simulink model "laboratory2_group2_ME_4212"  (R2024b)
settings: Solver=VariableStepAuto  StartTime=0.0  StopTime=Sim_Time  RelTol=1e-3
undefined symbols (not defined in the file): B1, B2, F, K1, K2, M1, M2
settings Model: Creator=karltzu  LastModifiedBy=karltzu

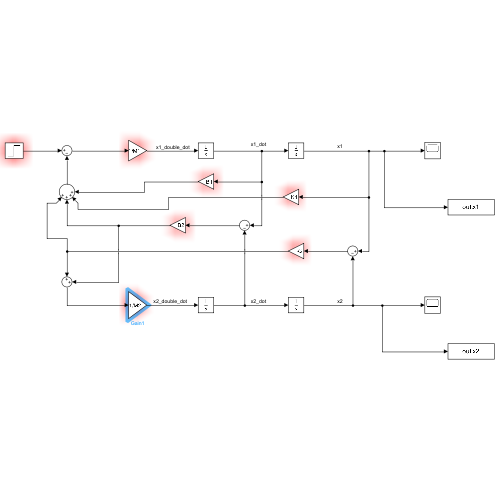
[thumbnail: Simulink's stored preview of the top-level diagram]
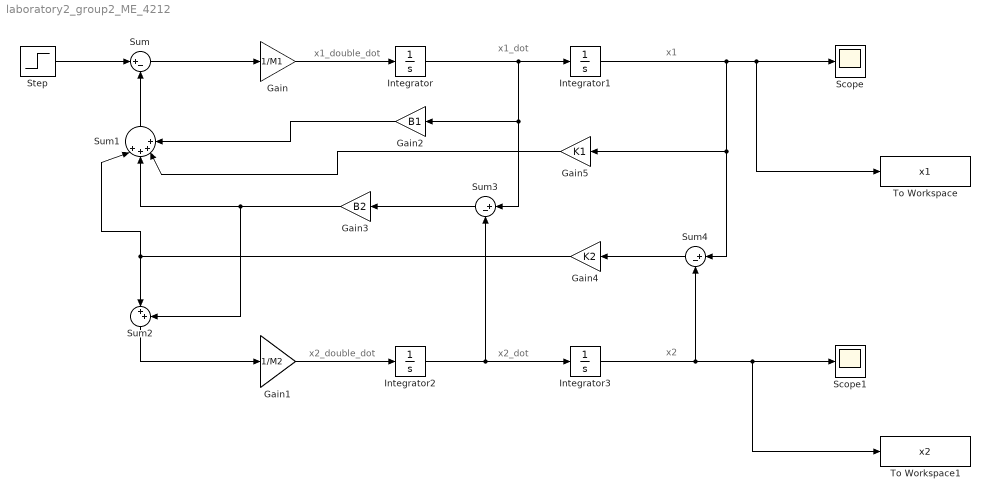
== system laboratory2_group2_ME_4212 ==
  note: x1_double_dot
  note: x2_double_dot
  note: x2_dot
  note: x1_dot
  note: x1
  note: x2
  Gain : Gain  Gain=1/M1
  Gain1 : Gain  Gain=1/M2
  Gain2 : Gain  Gain=B1
  Gain3 : Gain  Gain=B2
  Gain4 : Gain  Gain=K2
  Gain5 : Gain  Gain=K1
  Integrator{,1..3} (4 alike) : Integrator
  Scope : Scope
  Scope1 : Scope
  Step : Step  After=F  SampleTime=0
  Sum : Sum  Inputs=|+-
  Sum1 : Sum  Inputs=|++++
  Sum2 : Sum  Inputs=|++
  Sum3 : Sum  Inputs=|+-
  Sum4 : Sum  Inputs=|+-
  To Workspace : ToWorkspace  VariableName=x1  SaveFormat=Timeseries  SampleTime=-1
  To Workspace1 : ToWorkspace  VariableName=x2  SaveFormat=Timeseries  SampleTime=-1
  wires:
  Step/1 -> Sum/1
  Sum/1 -> Gain/1
  Gain/1 -> Integrator/1
  Integrator/1 -> Gain2/1, Sum3/1, Integrator1/1
  Integrator2/1 -> Sum3/2, Integrator3/1
  Integrator1/1 -> To Workspace/1, Scope/1, Gain5/1, Sum4/1
  Integrator3/1 -> To Workspace1/1, Scope1/1, Sum4/2
  Gain1/1 -> Integrator2/1
  Sum1/1 -> Sum/2
  Sum3/1 -> Gain3/1
  Sum4/1 -> Gain4/1
  Gain4/1 -> Sum2/1, Sum1/1
  Gain3/1 -> Sum2/2, Sum1/2
  Gain5/1 -> Sum1/3
  Gain2/1 -> Sum1/4
  Sum2/1 -> Gain1/1
